simulink model "ME655_project"  (R2023b)
settings: Solver=FixedStepAuto  StartTime=0.0  StopTime=60.0  FixedStep=.003  RelTol=1e-3
values from neighbouring files (symbols this model uses):
  A = [1 T; 0 1]    [ME655_project_Matlab_code.m]
  dt_active_control = 10    [ME655_project_Matlab_code.m]
  H = eye(2)    [ME655_project_Matlab_code.m]
  h = 2.5*N    (= 200)    [ME655_project_Matlab_code.m]
  K = Sp * C * inv(Sh)    [ME655_project_Matlab_code.m]
  k = -K * RhipAvg' + LhipAvg'    [ME655_project_Matlab_code.m]
  lambda = .95    (= 0.95)    [ME655_project_Matlab_code.m]
  Lhip_pos0 = Lhip_pos(1)    [ME655_project_Matlab_code.m]
  Lhip_vel0 = Lhip_vel(1)    [ME655_project_Matlab_code.m]
  M = 6    [ME655_project_Matlab_code.m]
  N = 80    [ME655_project_Matlab_code.m]
  nu = .5    (= 0.5)    [ME655_project_Matlab_code.m]
  Q = G * G' * var(Lhip_acc(train_indices))    [ME655_project_Matlab_code.m]
  R = diag([var(Lhip_pred(:, 1) - Lhip_pos_train), var(Lhip_pred(:, 2) - Lhip_vel_train)])    [ME655_project_Matlab_code.m]
  t_start = 5.0    (= 5)    [ME655_project_Matlab_code.m]
  Tau_h_max = 30    [ME655_project_Matlab_code.m]
undefined symbols (not defined in the file or in its folder): Bh, g, IHC, IRC, Kh, LH, LR, mH, mR, theta_0, theta_d0
settings Model: Creator=Damiano  LastModifiedBy=Mihir
settings SolverCC: AlgebraicLoopSolver=TrustRegion
settings DataIOCC: ReturnWorkspaceOutputs=off
settings DebuggingCC: UnconnectedInputMsg=warning  UnconnectedOutputMsg=warning  UnconnectedLineMsg=warning  ArithmeticOperatorsInVariantConditions=warning
settings ModelReferenceCC: EnableRefExpFcnMdlSchedulingChecks=on
settings SFSimCC: SimUseLocalCustomCode=off  CustomCodeUndefinedFunction=UseInterfaceOnly
settings RTWCC: RTWUseLocalCustomCode=off  DLArmComputeVersion=19.05
settings CodeAppCC: StateflowObjectComments=on

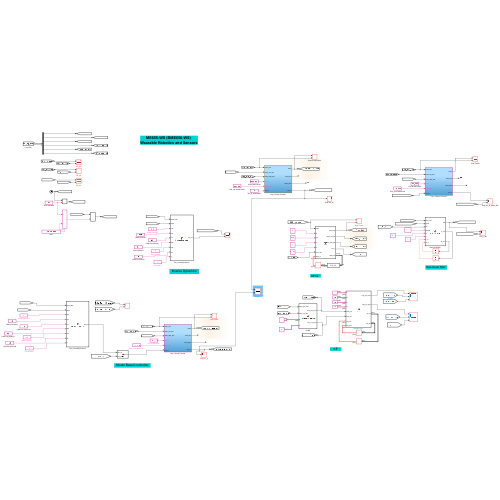
[thumbnail: Simulink's stored preview of the top-level diagram]
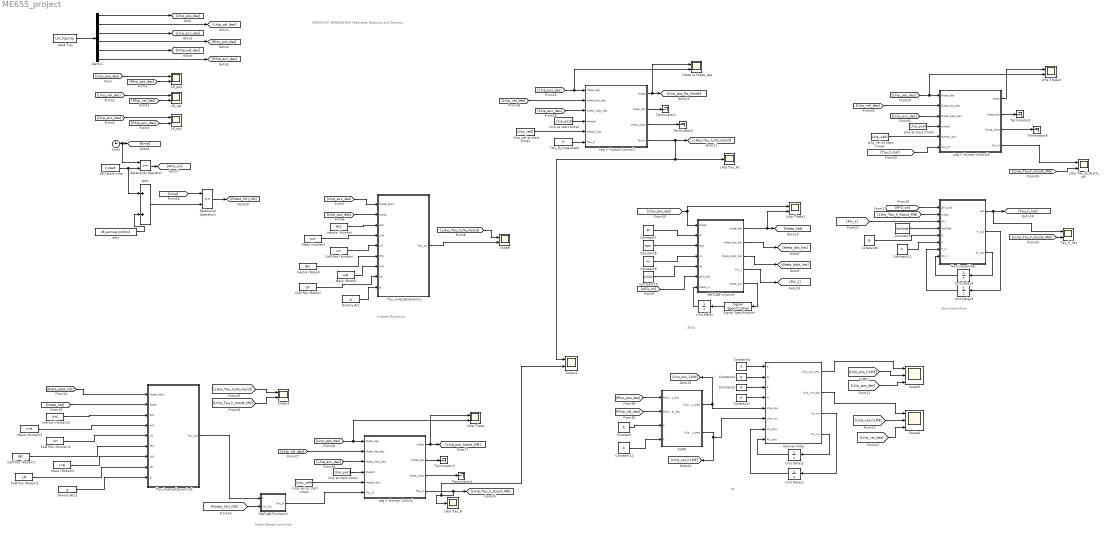
== system ME655_project ==
  note: ME655-WS (BME656-WS)
      | Wearable Robotics and Sensors
  note: AFOs
  note: Inverse Dynamics
  note: Model Based controller
  note: KF
  note: Non-linear filter
  AFO start time : Constant  Value=t_start
  Add : Sum
  CLME : MATLAB Function  TreatAsAtomicUnit=on
  Clock : Clock
  CoM Pos (Human) : Constant  Value=LH
  CoM Pos (Human)2 : Constant  Value=LH
  CoM Pos (Robot) : Constant  Value=LR
  CoM Pos (Robot)1 : Constant  Value=IRC
  CoM Pos (Robot)2 : Constant  Value=LR
  Constant : Constant  Value=K
  Constant1 : Constant  Value=H
  Constant10 : Constant  Value=0.003
  Constant11 : Constant  Value=h
  Constant12 : Constant  Value=k
  Constant2 : Constant  Value=R
  Constant3 : Constant  Value=Q
  Constant4 : Constant  Value=A
  Constant5 : Constant  Value=lambda
  Constant6 : Constant  Value=N
  Constant7 : Constant  Value=M
  Constant8 : Constant  Value=eps
  Constant9 : Constant  Value=nu
  Demux : Demux  Outputs=6
  Gravity Acc : Constant  Value=g
  Gravity Acc2 : Constant  Value=g
  Inertia (Human) : Constant  Value=IHC
  Inertia (Human)2 : Constant  Value=IHC
  Inertia (Robot) : Constant  Value=IRC
  Kalman Filter : MATLAB Function  TreatAsAtomicUnit=on
  LHip Tau_H : Scope
  LHip Tau_H1 : Scope
  LHip Tau_H_Assist_MF : Scope  NumInputPorts=2
  LHip Theta : Scope  NumInputPorts=2
  LHip Theta1 : Scope  NumInputPorts=2
  LHip Theta3 : Scope  NumInputPorts=2
  "LR_acc " : Scope  NumInputPorts=2
  LR_pos : Scope  NumInputPorts=2
  LR_vel : Scope  NumInputPorts=2
  Leg + Human Control : Subsystem
  Leg + Human Control1 : Subsystem
  Leg + Human Control2 : Subsystem
  Lhip at start time1 : Constant  Value=Lhip_pos0
  Lhip at start time2 : Constant  Value=Lhip_pos0
  Lhip at start time3 : Constant  Value=Lhip_pos0
  Lhip_vel at start time1 : Constant  Value=Lhip_vel0
  Lhip_vel at start time2 : Constant  Value=Lhip_vel0
  Lhip_vel at start time3 : Constant  Value=Lhip_vel0
  Load Traj : FromWorkspace  VariableName=LH_hip_traj
  MATLAB Function : MATLAB Function  TreatAsAtomicUnit=on
  MATLAB Function1 : MATLAB Function  TreatAsAtomicUnit=on
  Mass (Human) : Constant  Value=mH
  Mass (Human)2 : Constant  Value=mH
  Mass (Robot) : Constant  Value=mR
  Mass (Robot)2 : Constant  Value=mR
  NonLinearFilter : MATLAB Function  TreatAsAtomicUnit=on
  Relational Operator : RelationalOperator  OutDataTypeStr=boolean  RndMeth=Simplest  InputSameDT=off
  Relational Operator1 : RelationalOperator  OutDataTypeStr=boolean  RndMeth=Simplest  InputSameDT=off
  Scope : Scope  NumInputPorts=2
  Scope1 : Scope  NumInputPorts=2
  Scope3 : Scope  NumInputPorts=2
  Scope5 : Scope  NumInputPorts=3
  Scope6 : Scope  NumInputPorts=3
  Signal Specification : SignalSpecification  Dimensions=[1,14]
  Tau_InverseDynamics : MATLAB Function  TreatAsAtomicUnit=on
  Tau_InverseDynamics2 : MATLAB Function  TreatAsAtomicUnit=on
  Tau_R_Unassisted : Constant  Value=0
  Tau_h_hat : Scope  NumInputPorts=2
  Terminator{1..6} (6 alike) : Terminator
  Unit Delay : UnitDelay  InitialCondition=[[pi/2,pi/2,pi/2,pi/2,pi/2,pi/2],[0,0,0,0,0,0], 3*pi/2, 0]  SampleTime=-1  HasFrameUpgradeWarning=on
  Unit Delay1 : UnitDelay  InitialCondition=eye(2)  SampleTime=-1  HasFrameUpgradeWarning=on
  Unit Delay2 : UnitDelay  InitialCondition=[0;0]  SampleTime=-1  HasFrameUpgradeWarning=on
  Unit Delay3 : UnitDelay  InitialCondition=1  SampleTime=-1  HasFrameUpgradeWarning=on
  Unit Delay4 : UnitDelay  SampleTime=-1  HasFrameUpgradeWarning=on
  theta vs theta_des : Scope  NumInputPorts=2
  zero : Constant  Value=dt_active_control
  wires:
  Load Traj/1 -> Demux/1
  Demux/6 -> [Rhip_acc_des]
  Demux/4 -> [Rhip_pos_des]
  Demux/5 -> [Rhip_vel_des]
  [Lhip_pos_des] -> LR_pos/1
  [Rhip_pos_des] -> LR_pos/2
  [Lhip_vel_des] -> LR_vel/1
  [Rhip_vel_des] -> LR_vel/2
  [Lhip_acc_des] -> "LR_acc "/1
  [Rhip_acc_des] -> "LR_acc "/2
  Clock/1 -> Relational Operator/1, [time]
  Relational Operator/1 -> [AFO_on]
  [time] -> Relational Operator1/1
  AFO start time/1 -> Add/1, Relational Operator/2
  Add/1 -> Relational Operator1/2
  zero/1 -> Add/2
  [Lhip_acc_des] -> Leg + Human Control/3(theta_ddot_des)
  Leg + Human Control/3(theta_ddot) -> Terminator4/1
  Lhip_vel at start time1/1 -> Leg + Human Control/5(theta0_dot)
  Leg + Human Control/2(theta_dot) -> Terminator3/1
  [Lhip_vel_des] -> Leg + Human Control/2(theta_dot_des)
  Lhip at start time1/1 -> Leg + Human Control/4(theta0)
  Leg + Human Control/1(theta) -> LHip Theta/1, [Lhip_pos_Assist_MB]
  Leg + Human Control/4(Tau_h) -> Scope1/2, LHip Tau_H/1, [LHip_Tau_h_Assist_MB]
  [Lhip_pos_des] -> Leg + Human Control/1(theta_des), LHip Theta/2
  Relational Operator1/1 -> [Robot_Ctrl_ON]
  Demux/1 -> [Lhip_pos_des]
  Demux/2 -> [Lhip_vel_des]
  Demux/3 -> [Lhip_acc_des]
  Inertia (Robot)/1 -> Tau_InverseDynamics/6(IRC)
  Gravity Acc/1 -> Tau_InverseDynamics/9(g)
  Mass (Robot)/1 -> Tau_InverseDynamics/7(mR)
  Inertia (Human)/1 -> Tau_InverseDynamics/3(IHC)
  Mass (Human)/1 -> Tau_InverseDynamics/4(mH)
  CoM Pos (Robot)/1 -> Tau_InverseDynamics/8(LR)
  CoM Pos (Human)/1 -> Tau_InverseDynamics/5(LH)
  [Lhip_pos_des] -> Tau_InverseDynamics/2(theta)
  [Lhip_acc_des] -> Tau_InverseDynamics/1(theta_ddot)
  [LHip_Tau_h_No_Assist] -> Scope/1
  MATLAB Function/2(theta_dot_hat) -> [theta_dot_hat]
  MATLAB Function/1(theta_hat) -> [theta_hat], LHip Theta1/2
  MATLAB Function/3(theta_ddot_hat) -> [theta_ddot_hat]
  [AFO_on] -> MATLAB Function/6(AFO_ON)
  Signal Specification/1 -> Unit Delay/1
  [Lhip_pos_des] -> LHip Theta1/1, MATLAB Function/1(theta)
  Constant7/1 -> MATLAB Function/2(M)
  Constant8/1 -> MATLAB Function/3(eps)
  Constant10/1 -> MATLAB Function/5(dt)
  Constant9/1 -> MATLAB Function/4(nu)
  Tau_InverseDynamics/1(Tau_tot) -> Scope/2
  MATLAB Function/5(state_out) -> Signal Specification/1
  Unit Delay/1 -> MATLAB Function/7(state_in)
  [LHip_Tau_h_Assist_MB] -> Scope3/2
  Mass (Robot)2/1 -> Tau_InverseDynamics2/7(mR)
  Tau_InverseDynamics2/1(Tau_tot) -> MATLAB Function1/1(Tau_tot)
  Mass (Human)2/1 -> Tau_InverseDynamics2/4(mH)
  Gravity Acc2/1 -> Tau_InverseDynamics2/9(g)
  Inertia (Human)2/1 -> Tau_InverseDynamics2/3(IHC)
  [theta_hat] -> Tau_InverseDynamics2/2(theta)
  CoM Pos (Human)2/1 -> Tau_InverseDynamics2/5(LH)
  [theta_ddot_hat] -> Tau_InverseDynamics2/1(theta_ddot)
  CoM Pos (Robot)2/1 -> Tau_InverseDynamics2/8(LR)
  CoM Pos (Robot)1/1 -> Tau_InverseDynamics2/6(IRC)
  [LHip_Tau_h_No_Assist] -> Scope3/1
  Constant2/1 -> Kalman Filter/3(R)
  Constant3/1 -> Kalman Filter/2(Q)
  Constant4/1 -> Kalman Filter/1(A)
  Kalman Filter/2(Lhip_vel_des) -> Scope6/1
  Kalman Filter/4(Pk_nxt) -> Unit Delay1/1
  Kalman Filter/1(Lhip_pos_des) -> Scope5/1
  Unit Delay2/1 -> Kalman Filter/7(xk_prev)
  [Lhip_vel_des] -> Scope6/3
  [Lhip_pos_CLME] -> Scope5/2
  [Lhip_vel_CLME] -> Scope6/2
  [Lhip_pos_des] -> Scope5/3
  Constant1/1 -> Kalman Filter/4(H)
  Kalman Filter/3(xk_nxt) -> Unit Delay2/1
  Unit Delay1/1 -> Kalman Filter/8(Pk_prev)
  MATLAB Function1/1(Tau_R) -> Leg + Human Control/6(Tau_R)
  Leg + Human Control1/3(theta_ddot) -> Terminator2/1
  Leg + Human Control1/2(theta_dot) -> Terminator1/1
  [Lhip_pos_des] -> Leg + Human Control1/1(theta_des), theta vs theta_des/2
  [Lhip_vel_des] -> Leg + Human Control1/2(theta_dot_des)
  Lhip_vel at start time2/1 -> Leg + Human Control1/5(theta0_dot)
  Leg + Human Control1/4(Tau_h) -> LHip Tau_H1/1, Scope1/1, [LHip_Tau_h_No_Assist]
  Lhip at start time2/1 -> Leg + Human Control1/4(theta0)
  Tau_R_Unassisted/1 -> Leg + Human Control1/6(Tau_R)
  [Lhip_acc_des] -> Leg + Human Control1/3(theta_ddot_des)
  Leg + Human Control1/1(theta) -> theta vs theta_des/1, [Lhip_pos_No_Assist]
  [Robot_Ctrl_ON] -> MATLAB Function1/2(Ctrl_On)
  MATLAB Function/4(Phi_1) -> [Phi_1]
  NonLinearFilter/1(est) -> Tau_h_hat/1, [Tau_h_hat]
  NonLinearFilter/3(W_out) -> Unit Delay4/1
  [AFO_on] -> NonLinearFilter/1(AFO_ON)
  Unit Delay4/1 -> NonLinearFilter/8(W_in)
  Constant11/1 -> NonLinearFilter/6(h)
  NonLinearFilter/2(P_out) -> Unit Delay3/1
  Constant6/1 -> NonLinearFilter/5(N)
  Unit Delay3/1 -> NonLinearFilter/7(P_in)
  Constant5/1 -> NonLinearFilter/4(lambda)
  [LHip_Tau_h_Assist_MB] -> NonLinearFilter/2(meas)
  [Phi_1] -> NonLinearFilter/3(phi)
  [Lhip_vel_des] -> Leg + Human Control2/2(theta_dot_des)
  Leg + Human Control2/2(theta_dot) -> Terminator5/1
  [Lhip_acc_des] -> Leg + Human Control2/3(theta_ddot_des)
  Leg + Human Control2/1(theta) -> LHip Theta3/1
  Lhip_vel at start time3/1 -> Leg + Human Control2/5(theta0_dot)
  Lhip at start time3/1 -> Leg + Human Control2/4(theta0)
  Leg + Human Control2/4(Tau_h) -> LHip Tau_H_Assist_MF/1
  [Tau_h_hat] -> Leg + Human Control2/6(Tau_R)
  Leg + Human Control2/3(theta_ddot) -> Terminator6/1
  [Lhip_pos_des] -> Leg + Human Control2/1(theta_des), LHip Theta3/2
  [LHip_Tau_h_Assist_MB] -> LHip Tau_H_Assist_MF/2
  [Rhip_vel_des] -> CLME/2(Rhip_vel_des)
  [Rhip_pos_des] -> CLME/1(Rhip_pos_des)
  Constant/1 -> CLME/3(K)
  Constant12/1 -> CLME/4(k)
  CLME/1(Lhip_pos_pred) -> [Lhip_pos_CLME], Kalman Filter/5(Lhip_pos)
  CLME/2(Lhip_vel_pred) -> [Lhip_vel_CLME], Kalman Filter/6(Lhip_vel)
  [LHip_Tau_h_Assist_MB] -> Tau_h_hat/2

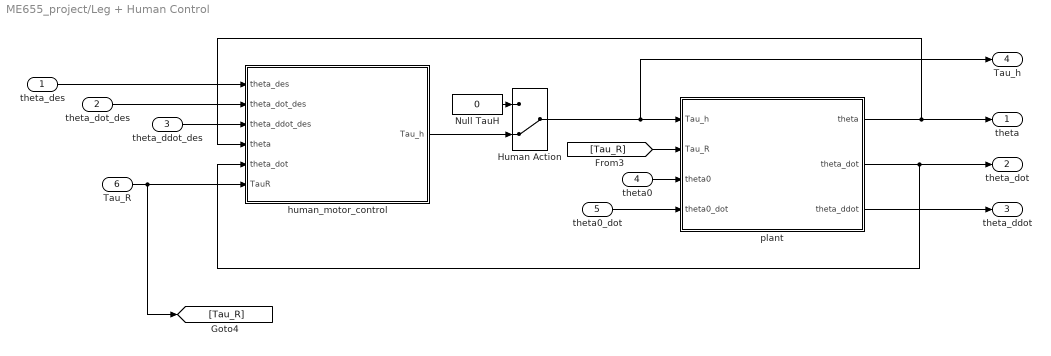
== system ME655_project/Leg + Human Control ==
  theta_des : Inport
  theta_dot_des : Inport  Port=2
  theta_ddot_des : Inport  Port=3
  theta0 : Inport  Port=4
  theta0_dot : Inport  Port=5
  Tau_R : Inport  Port=6
  Human Action : ManualSwitch  CurrentSetting=0
  Null TauH : Constant  Value=0
  human_motor_control : Subsystem
  plant : Subsystem
  theta : Outport  PortDimensions=[1,1]  VectorParamsAs1DForOutWhenUnconnected=off
  theta_dot : Outport  Port=2  PortDimensions=[1,1]  VectorParamsAs1DForOutWhenUnconnected=off
  theta_ddot : Outport  Port=3  PortDimensions=[1,1]  VectorParamsAs1DForOutWhenUnconnected=off
  Tau_h : Outport  Port=4  PortDimensions=[1,1]  VectorParamsAs1DForOutWhenUnconnected=off
  wires:
  theta_des/1 -> human_motor_control/1(theta_des)
  theta_dot_des/1 -> human_motor_control/2(theta_dot_des)
  theta0/1 -> plant/3(theta0)
  theta0_dot/1 -> plant/4(theta0_dot)
  [Tau_R] -> plant/2(Tau_R)
  plant/1(theta) -> theta/1, human_motor_control/4(theta)
  plant/2(theta_dot) -> human_motor_control/5(theta_dot), theta_dot/1
  plant/3(theta_ddot) -> theta_ddot/1
  theta_ddot_des/1 -> human_motor_control/3(theta_ddot_des)
  human_motor_control/1(Tau_h) -> Human Action/2
  Human Action/1 -> Tau_h/1, plant/1(Tau_h)
  Null TauH/1 -> Human Action/1
  Tau_R/1 -> [Tau_R], human_motor_control/6(TauR)

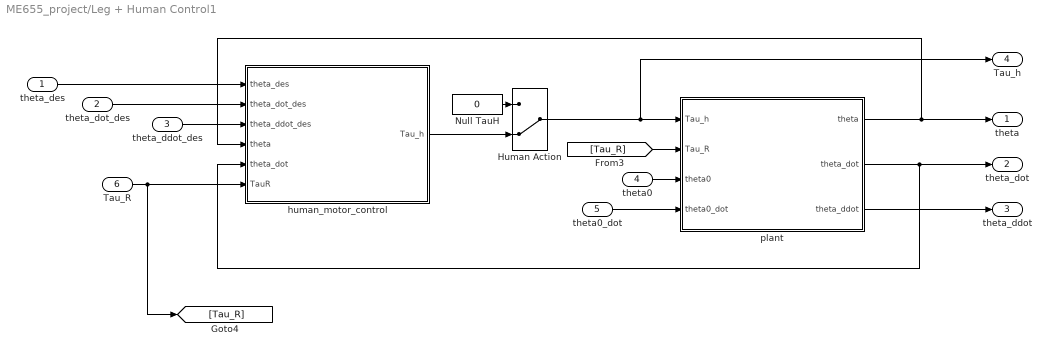
== system ME655_project/Leg + Human Control1 ==
  theta_des : Inport
  theta_dot_des : Inport  Port=2
  theta_ddot_des : Inport  Port=3
  theta0 : Inport  Port=4
  theta0_dot : Inport  Port=5
  Tau_R : Inport  Port=6
  Human Action : ManualSwitch  CurrentSetting=0
  Null TauH : Constant  Value=0
  human_motor_control : Subsystem
  plant : Subsystem
  theta : Outport  PortDimensions=[1,1]  VectorParamsAs1DForOutWhenUnconnected=off
  theta_dot : Outport  Port=2  PortDimensions=[1,1]  VectorParamsAs1DForOutWhenUnconnected=off
  theta_ddot : Outport  Port=3  PortDimensions=[1,1]  VectorParamsAs1DForOutWhenUnconnected=off
  Tau_h : Outport  Port=4  PortDimensions=[1,1]  VectorParamsAs1DForOutWhenUnconnected=off
  wires:
  theta_des/1 -> human_motor_control/1(theta_des)
  theta_dot_des/1 -> human_motor_control/2(theta_dot_des)
  theta0/1 -> plant/3(theta0)
  theta0_dot/1 -> plant/4(theta0_dot)
  [Tau_R] -> plant/2(Tau_R)
  plant/1(theta) -> theta/1, human_motor_control/4(theta)
  plant/2(theta_dot) -> human_motor_control/5(theta_dot), theta_dot/1
  plant/3(theta_ddot) -> theta_ddot/1
  theta_ddot_des/1 -> human_motor_control/3(theta_ddot_des)
  human_motor_control/1(Tau_h) -> Human Action/2
  Human Action/1 -> Tau_h/1, plant/1(Tau_h)
  Null TauH/1 -> Human Action/1
  Tau_R/1 -> [Tau_R], human_motor_control/6(TauR)

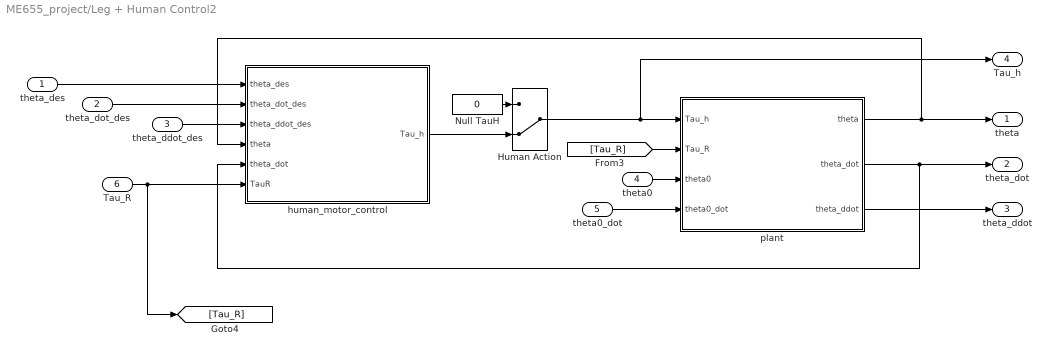
== system ME655_project/Leg + Human Control2 ==
  theta_des : Inport
  theta_dot_des : Inport  Port=2
  theta_ddot_des : Inport  Port=3
  theta0 : Inport  Port=4
  theta0_dot : Inport  Port=5
  Tau_R : Inport  Port=6
  Human Action : ManualSwitch  CurrentSetting=0
  Null TauH : Constant  Value=0
  human_motor_control : Subsystem
  plant : Subsystem
  theta : Outport  PortDimensions=[1,1]  VectorParamsAs1DForOutWhenUnconnected=off
  theta_dot : Outport  Port=2  PortDimensions=[1,1]  VectorParamsAs1DForOutWhenUnconnected=off
  theta_ddot : Outport  Port=3  PortDimensions=[1,1]  VectorParamsAs1DForOutWhenUnconnected=off
  Tau_h : Outport  Port=4  PortDimensions=[1,1]  VectorParamsAs1DForOutWhenUnconnected=off
  wires:
  theta_des/1 -> human_motor_control/1(theta_des)
  theta_dot_des/1 -> human_motor_control/2(theta_dot_des)
  theta0/1 -> plant/3(theta0)
  theta0_dot/1 -> plant/4(theta0_dot)
  [Tau_R] -> plant/2(Tau_R)
  plant/1(theta) -> theta/1, human_motor_control/4(theta)
  plant/2(theta_dot) -> human_motor_control/5(theta_dot), theta_dot/1
  plant/3(theta_ddot) -> theta_ddot/1
  theta_ddot_des/1 -> human_motor_control/3(theta_ddot_des)
  human_motor_control/1(Tau_h) -> Human Action/2
  Human Action/1 -> Tau_h/1, plant/1(Tau_h)
  Null TauH/1 -> Human Action/1
  Tau_R/1 -> [Tau_R], human_motor_control/6(TauR)

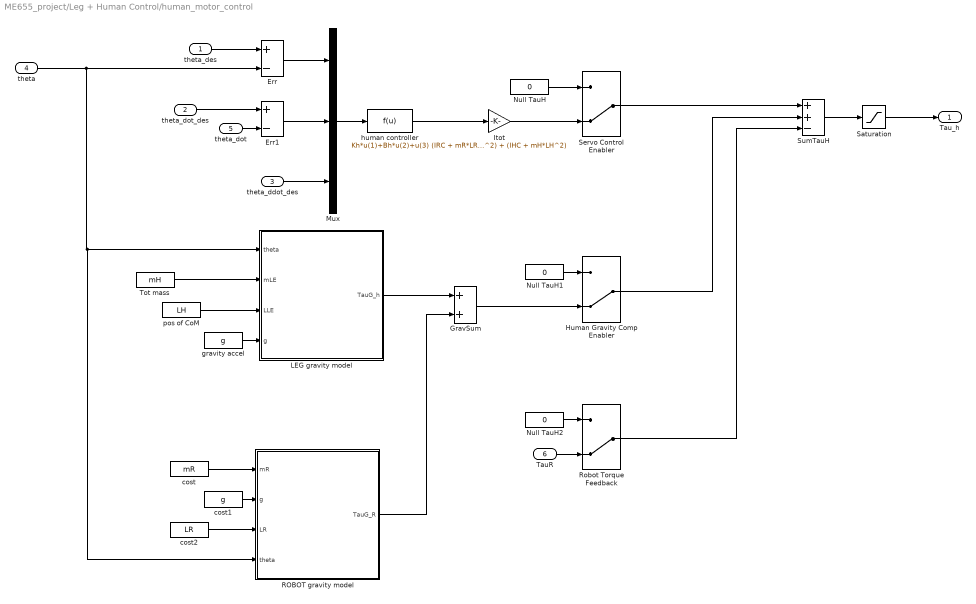
== system ME655_project/Leg + Human Control/human_motor_control ==
  theta_des : Inport
  theta_dot_des : Inport  Port=2
  theta_ddot_des : Inport  Port=3
  theta : Inport  Port=4
  theta_dot : Inport  Port=5
  TauR : Inport  Port=6
  Err : Sum  Inputs=+-
  Err1 : Sum  Inputs=+-
  GravSum : Sum
  Human Gravity Comp Enabler : ManualSwitch  CurrentSetting=0
  Itot : Gain  Gain=(IRC + mR*LR^2) + (IHC + mH*LH^2)
  LEG gravity model : MATLAB Function  TreatAsAtomicUnit=on
  Mux : Mux  Inputs=3
  Null TauH : Constant  Value=0
  Null TauH1 : Constant  Value=0
  Null TauH2 : Constant  Value=0
  ROBOT gravity model : MATLAB Function  TreatAsAtomicUnit=on
  Robot Torque Feedback : ManualSwitch  CurrentSetting=0
  Saturation : Saturate  UpperLimit=Tau_h_max  LowerLimit=-Tau_h_max
  Servo Control Enabler : ManualSwitch  CurrentSetting=0
  SumTauH : Sum  Inputs=++-
  Tot mass : Constant  Value=mH
  cost : Constant  Value=mR
  cost1 : Constant  Value=g
  cost2 : Constant  Value=LR
  gravity accel : Constant  Value=g
  human controller : Fcn  Expr=Kh*u(1)+Bh*u(2)+u(3)
  pos of CoM : Constant  Value=LH
  Tau_h : Outport  PortDimensions=[1,1]  VectorParamsAs1DForOutWhenUnconnected=off
  wires:
  theta_des/1 -> Err/1
  theta_dot_des/1 -> Err1/1
  theta_dot/1 -> Err1/2
  Err/1 -> Mux/1
  Err1/1 -> Mux/2
  Mux/1 -> human controller/1
  theta_ddot_des/1 -> Mux/3
  gravity accel/1 -> LEG gravity model/4(g)
  Tot mass/1 -> LEG gravity model/2(mLE)
  pos of CoM/1 -> LEG gravity model/3(LLE)
  Null TauH/1 -> Servo Control Enabler/1
  Null TauH1/1 -> Human Gravity Comp Enabler/1
  Human Gravity Comp Enabler/1 -> SumTauH/2
  SumTauH/1 -> Saturation/1
  human controller/1 -> Itot/1
  Servo Control Enabler/1 -> SumTauH/1
  Saturation/1 -> Tau_h/1
  Itot/1 -> Servo Control Enabler/2
  Null TauH2/1 -> Robot Torque Feedback/1
  TauR/1 -> Robot Torque Feedback/2
  Robot Torque Feedback/1 -> SumTauH/3
  theta/1 -> ROBOT gravity model/4(theta), LEG gravity model/1(theta), Err/2
  ROBOT gravity model/1(TauG_R) -> GravSum/2
  cost2/1 -> ROBOT gravity model/3(LR)
  cost/1 -> ROBOT gravity model/1(mR)
  cost1/1 -> ROBOT gravity model/2(g)
  LEG gravity model/1(TauG_h) -> GravSum/1
  GravSum/1 -> Human Gravity Comp Enabler/2

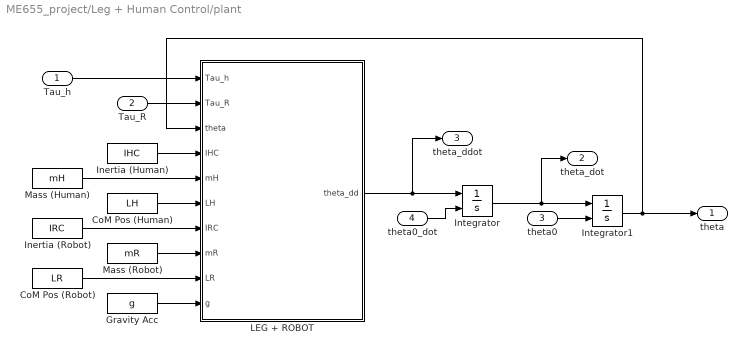
== system ME655_project/Leg + Human Control/plant ==
  Tau_h : Inport
  Tau_R : Inport  Port=2
  theta0 : Inport  Port=3
  theta0_dot : Inport  Port=4
  CoM Pos (Human) : Constant  Value=LH
  CoM Pos (Robot) : Constant  Value=LR
  Gravity Acc : Constant  Value=g
  Inertia (Human) : Constant  Value=IHC
  Inertia (Robot) : Constant  Value=IRC
  Integrator : Integrator  InitialConditionSource=external  InitialCondition=theta_d0
  Integrator1 : Integrator  InitialConditionSource=external  InitialCondition=theta_0
  LEG + ROBOT : MATLAB Function  TreatAsAtomicUnit=on
  Mass (Human) : Constant  Value=mH
  Mass (Robot) : Constant  Value=mR
  theta : Outport  PortDimensions=[1,1]  VectorParamsAs1DForOutWhenUnconnected=off
  theta_dot : Outport  Port=2  PortDimensions=[1,1]  VectorParamsAs1DForOutWhenUnconnected=off
  theta_ddot : Outport  Port=3  PortDimensions=[1,1]  VectorParamsAs1DForOutWhenUnconnected=off
  wires:
  Tau_h/1 -> LEG + ROBOT/1(Tau_h)
  Tau_R/1 -> LEG + ROBOT/2(Tau_R)
  LEG + ROBOT/1(theta_dd) -> theta_ddot/1, Integrator/1
  Integrator/1 -> theta_dot/1, Integrator1/1
  theta0_dot/1 -> Integrator/2
  theta0/1 -> Integrator1/2
  Integrator1/1 -> LEG + ROBOT/3(theta), theta/1
  Inertia (Human)/1 -> LEG + ROBOT/4(IHC)
  Mass (Human)/1 -> LEG + ROBOT/5(mH)
  CoM Pos (Human)/1 -> LEG + ROBOT/6(LH)
  Gravity Acc/1 -> LEG + ROBOT/10(g)
  Mass (Robot)/1 -> LEG + ROBOT/8(mR)
  CoM Pos (Robot)/1 -> LEG + ROBOT/9(LR)
  Inertia (Robot)/1 -> LEG + ROBOT/7(IRC)

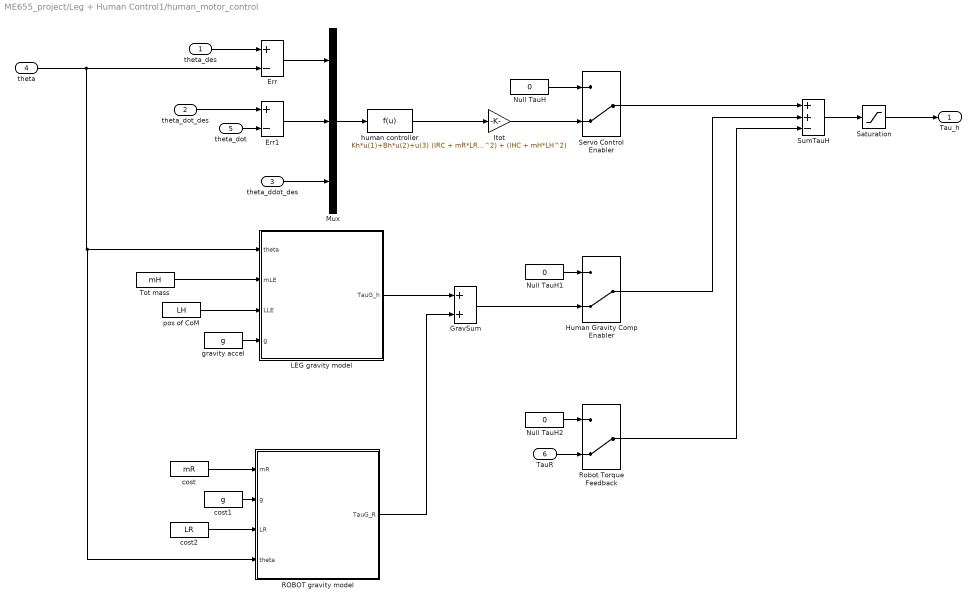
== system ME655_project/Leg + Human Control1/human_motor_control ==
  theta_des : Inport
  theta_dot_des : Inport  Port=2
  theta_ddot_des : Inport  Port=3
  theta : Inport  Port=4
  theta_dot : Inport  Port=5
  TauR : Inport  Port=6
  Err : Sum  Inputs=+-
  Err1 : Sum  Inputs=+-
  GravSum : Sum
  Human Gravity Comp Enabler : ManualSwitch  CurrentSetting=0
  Itot : Gain  Gain=(IRC + mR*LR^2) + (IHC + mH*LH^2)
  LEG gravity model : MATLAB Function  TreatAsAtomicUnit=on
  Mux : Mux  Inputs=3
  Null TauH : Constant  Value=0
  Null TauH1 : Constant  Value=0
  Null TauH2 : Constant  Value=0
  ROBOT gravity model : MATLAB Function  TreatAsAtomicUnit=on
  Robot Torque Feedback : ManualSwitch  CurrentSetting=0
  Saturation : Saturate  UpperLimit=Tau_h_max  LowerLimit=-Tau_h_max
  Servo Control Enabler : ManualSwitch  CurrentSetting=0
  SumTauH : Sum  Inputs=++-
  Tot mass : Constant  Value=mH
  cost : Constant  Value=mR
  cost1 : Constant  Value=g
  cost2 : Constant  Value=LR
  gravity accel : Constant  Value=g
  human controller : Fcn  Expr=Kh*u(1)+Bh*u(2)+u(3)
  pos of CoM : Constant  Value=LH
  Tau_h : Outport  PortDimensions=[1,1]  VectorParamsAs1DForOutWhenUnconnected=off
  wires:
  theta_des/1 -> Err/1
  theta_dot_des/1 -> Err1/1
  theta_dot/1 -> Err1/2
  Err/1 -> Mux/1
  Err1/1 -> Mux/2
  Mux/1 -> human controller/1
  theta_ddot_des/1 -> Mux/3
  gravity accel/1 -> LEG gravity model/4(g)
  Tot mass/1 -> LEG gravity model/2(mLE)
  pos of CoM/1 -> LEG gravity model/3(LLE)
  Null TauH/1 -> Servo Control Enabler/1
  Null TauH1/1 -> Human Gravity Comp Enabler/1
  Human Gravity Comp Enabler/1 -> SumTauH/2
  SumTauH/1 -> Saturation/1
  human controller/1 -> Itot/1
  Servo Control Enabler/1 -> SumTauH/1
  Saturation/1 -> Tau_h/1
  Itot/1 -> Servo Control Enabler/2
  Null TauH2/1 -> Robot Torque Feedback/1
  TauR/1 -> Robot Torque Feedback/2
  Robot Torque Feedback/1 -> SumTauH/3
  theta/1 -> ROBOT gravity model/4(theta), LEG gravity model/1(theta), Err/2
  ROBOT gravity model/1(TauG_R) -> GravSum/2
  cost2/1 -> ROBOT gravity model/3(LR)
  cost/1 -> ROBOT gravity model/1(mR)
  cost1/1 -> ROBOT gravity model/2(g)
  LEG gravity model/1(TauG_h) -> GravSum/1
  GravSum/1 -> Human Gravity Comp Enabler/2

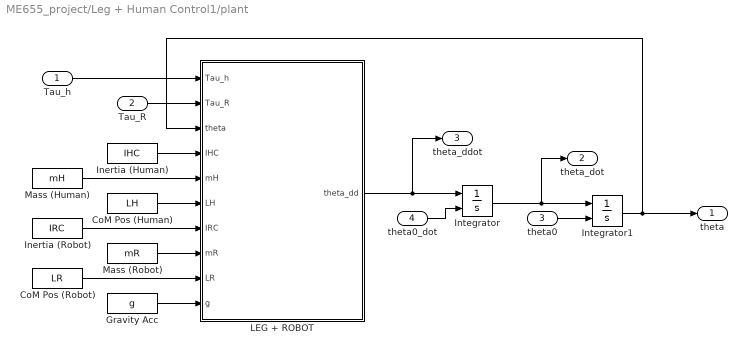
== system ME655_project/Leg + Human Control1/plant ==
  Tau_h : Inport
  Tau_R : Inport  Port=2
  theta0 : Inport  Port=3
  theta0_dot : Inport  Port=4
  CoM Pos (Human) : Constant  Value=LH
  CoM Pos (Robot) : Constant  Value=LR
  Gravity Acc : Constant  Value=g
  Inertia (Human) : Constant  Value=IHC
  Inertia (Robot) : Constant  Value=IRC
  Integrator : Integrator  InitialConditionSource=external  InitialCondition=theta_d0
  Integrator1 : Integrator  InitialConditionSource=external  InitialCondition=theta_0
  LEG + ROBOT : MATLAB Function  TreatAsAtomicUnit=on
  Mass (Human) : Constant  Value=mH
  Mass (Robot) : Constant  Value=mR
  theta : Outport  PortDimensions=[1,1]  VectorParamsAs1DForOutWhenUnconnected=off
  theta_dot : Outport  Port=2  PortDimensions=[1,1]  VectorParamsAs1DForOutWhenUnconnected=off
  theta_ddot : Outport  Port=3  PortDimensions=[1,1]  VectorParamsAs1DForOutWhenUnconnected=off
  wires:
  Tau_h/1 -> LEG + ROBOT/1(Tau_h)
  Tau_R/1 -> LEG + ROBOT/2(Tau_R)
  LEG + ROBOT/1(theta_dd) -> theta_ddot/1, Integrator/1
  Integrator/1 -> theta_dot/1, Integrator1/1
  theta0_dot/1 -> Integrator/2
  theta0/1 -> Integrator1/2
  Integrator1/1 -> LEG + ROBOT/3(theta), theta/1
  Inertia (Human)/1 -> LEG + ROBOT/4(IHC)
  Mass (Human)/1 -> LEG + ROBOT/5(mH)
  CoM Pos (Human)/1 -> LEG + ROBOT/6(LH)
  Gravity Acc/1 -> LEG + ROBOT/10(g)
  Mass (Robot)/1 -> LEG + ROBOT/8(mR)
  CoM Pos (Robot)/1 -> LEG + ROBOT/9(LR)
  Inertia (Robot)/1 -> LEG + ROBOT/7(IRC)

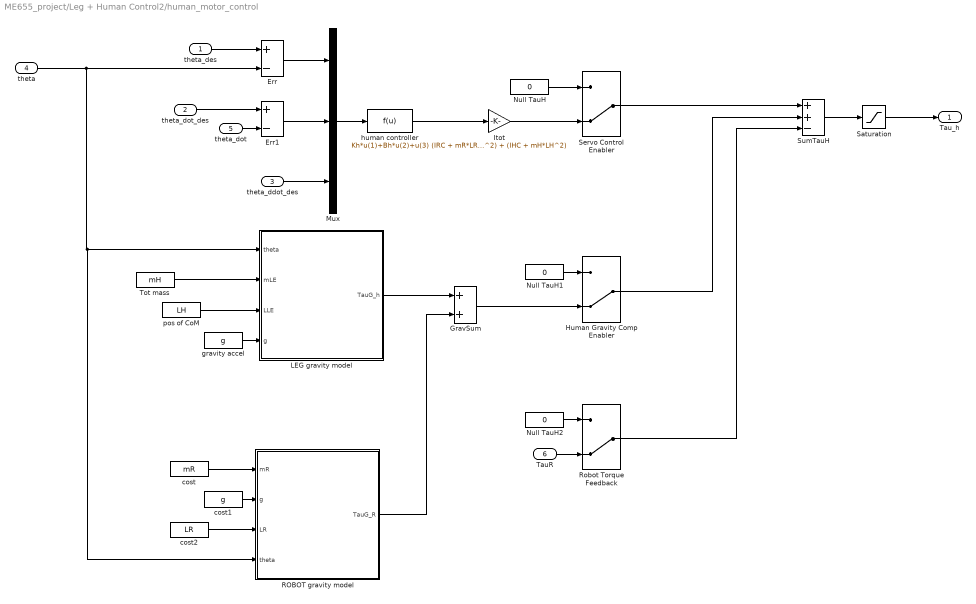
== system ME655_project/Leg + Human Control2/human_motor_control ==
  theta_des : Inport
  theta_dot_des : Inport  Port=2
  theta_ddot_des : Inport  Port=3
  theta : Inport  Port=4
  theta_dot : Inport  Port=5
  TauR : Inport  Port=6
  Err : Sum  Inputs=+-
  Err1 : Sum  Inputs=+-
  GravSum : Sum
  Human Gravity Comp Enabler : ManualSwitch  CurrentSetting=0
  Itot : Gain  Gain=(IRC + mR*LR^2) + (IHC + mH*LH^2)
  LEG gravity model : MATLAB Function  TreatAsAtomicUnit=on
  Mux : Mux  Inputs=3
  Null TauH : Constant  Value=0
  Null TauH1 : Constant  Value=0
  Null TauH2 : Constant  Value=0
  ROBOT gravity model : MATLAB Function  TreatAsAtomicUnit=on
  Robot Torque Feedback : ManualSwitch  CurrentSetting=0
  Saturation : Saturate  UpperLimit=Tau_h_max  LowerLimit=-Tau_h_max
  Servo Control Enabler : ManualSwitch  CurrentSetting=0
  SumTauH : Sum  Inputs=++-
  Tot mass : Constant  Value=mH
  cost : Constant  Value=mR
  cost1 : Constant  Value=g
  cost2 : Constant  Value=LR
  gravity accel : Constant  Value=g
  human controller : Fcn  Expr=Kh*u(1)+Bh*u(2)+u(3)
  pos of CoM : Constant  Value=LH
  Tau_h : Outport  PortDimensions=[1,1]  VectorParamsAs1DForOutWhenUnconnected=off
  wires:
  theta_des/1 -> Err/1
  theta_dot_des/1 -> Err1/1
  theta_dot/1 -> Err1/2
  Err/1 -> Mux/1
  Err1/1 -> Mux/2
  Mux/1 -> human controller/1
  theta_ddot_des/1 -> Mux/3
  gravity accel/1 -> LEG gravity model/4(g)
  Tot mass/1 -> LEG gravity model/2(mLE)
  pos of CoM/1 -> LEG gravity model/3(LLE)
  Null TauH/1 -> Servo Control Enabler/1
  Null TauH1/1 -> Human Gravity Comp Enabler/1
  Human Gravity Comp Enabler/1 -> SumTauH/2
  SumTauH/1 -> Saturation/1
  human controller/1 -> Itot/1
  Servo Control Enabler/1 -> SumTauH/1
  Saturation/1 -> Tau_h/1
  Itot/1 -> Servo Control Enabler/2
  Null TauH2/1 -> Robot Torque Feedback/1
  TauR/1 -> Robot Torque Feedback/2
  Robot Torque Feedback/1 -> SumTauH/3
  theta/1 -> ROBOT gravity model/4(theta), LEG gravity model/1(theta), Err/2
  ROBOT gravity model/1(TauG_R) -> GravSum/2
  cost2/1 -> ROBOT gravity model/3(LR)
  cost/1 -> ROBOT gravity model/1(mR)
  cost1/1 -> ROBOT gravity model/2(g)
  LEG gravity model/1(TauG_h) -> GravSum/1
  GravSum/1 -> Human Gravity Comp Enabler/2

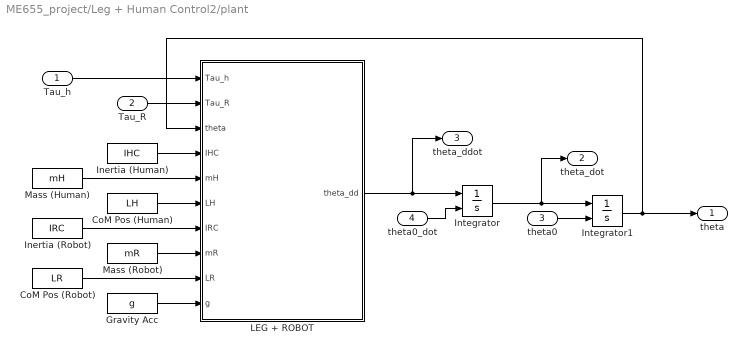
== system ME655_project/Leg + Human Control2/plant ==
  Tau_h : Inport
  Tau_R : Inport  Port=2
  theta0 : Inport  Port=3
  theta0_dot : Inport  Port=4
  CoM Pos (Human) : Constant  Value=LH
  CoM Pos (Robot) : Constant  Value=LR
  Gravity Acc : Constant  Value=g
  Inertia (Human) : Constant  Value=IHC
  Inertia (Robot) : Constant  Value=IRC
  Integrator : Integrator  InitialConditionSource=external  InitialCondition=theta_d0
  Integrator1 : Integrator  InitialConditionSource=external  InitialCondition=theta_0
  LEG + ROBOT : MATLAB Function  TreatAsAtomicUnit=on
  Mass (Human) : Constant  Value=mH
  Mass (Robot) : Constant  Value=mR
  theta : Outport  PortDimensions=[1,1]  VectorParamsAs1DForOutWhenUnconnected=off
  theta_dot : Outport  Port=2  PortDimensions=[1,1]  VectorParamsAs1DForOutWhenUnconnected=off
  theta_ddot : Outport  Port=3  PortDimensions=[1,1]  VectorParamsAs1DForOutWhenUnconnected=off
  wires:
  Tau_h/1 -> LEG + ROBOT/1(Tau_h)
  Tau_R/1 -> LEG + ROBOT/2(Tau_R)
  LEG + ROBOT/1(theta_dd) -> theta_ddot/1, Integrator/1
  Integrator/1 -> theta_dot/1, Integrator1/1
  theta0_dot/1 -> Integrator/2
  theta0/1 -> Integrator1/2
  Integrator1/1 -> LEG + ROBOT/3(theta), theta/1
  Inertia (Human)/1 -> LEG + ROBOT/4(IHC)
  Mass (Human)/1 -> LEG + ROBOT/5(mH)
  CoM Pos (Human)/1 -> LEG + ROBOT/6(LH)
  Gravity Acc/1 -> LEG + ROBOT/10(g)
  Mass (Robot)/1 -> LEG + ROBOT/8(mR)
  CoM Pos (Robot)/1 -> LEG + ROBOT/9(LR)
  Inertia (Robot)/1 -> LEG + ROBOT/7(IRC)

== matlab function ME655_project/Leg + Human Control2/human_motor_control/LEG gravity model ==
  data: theta input; mLE input; LLE input; TauG_h output; g input
function TauG_h   = HumanLegGravModel(theta,mLE,LLE,g)
% human gravity compensation term
TauG_h=mLE*g*LLE*sin(theta);

end

== matlab function ME655_project/Leg + Human Control/human_motor_control/LEG gravity model ==
  data: theta input; mLE input; LLE input; TauG_h output; g input
function TauG_h   = HumanLegGravModel(theta,mLE,LLE,g)
% human gravity compensation term
TauG_h=mLE*g*LLE*sin(theta);

end

== matlab function ME655_project/Leg + Human Control2/human_motor_control/ROBOT gravity model ==
  data: mR input; g input; LR input; theta input; TauG_R output
function TauG_R  = RobotGravModel(mR,g,LR,theta)

TauG_R=mR*g*LR*sin(theta);
% TauG_h=mLE*g*LLE*sin(theta);

end

== matlab function ME655_project/Tau_InverseDynamics2 ==
  data: theta_ddot input; Tau_tot output; theta input; IHC input; mH input; LH input; IRC input; mR input; LR input; g input
function Tau_tot = InverseDynamics(theta_ddot,theta,IHC,mH,LH,IRC,mR,LR,g)
Tau_tot = theta_ddot*((IRC + mR*LR^2)+(IHC + mH*LH^2)) + mH*g*LH*sin(theta) + mR*g*LR*sin(theta);

== matlab function ME655_project/Leg + Human Control/human_motor_control/ROBOT gravity model ==
  data: mR input; g input; LR input; theta input; TauG_R output
function TauG_R  = RobotGravModel(mR,g,LR,theta)

TauG_R=mR*g*LR*sin(theta);
% TauG_h=mLE*g*LLE*sin(theta);

end

== matlab function ME655_project/Leg + Human Control1/plant/LEG + ROBOT ==
  data: Tau_h input; Tau_R input; theta input; theta_dd output; IHC input; mH input; LH input; IRC input; mR input; LR input; g input
function theta_dd   = LegRobotModel(Tau_h,Tau_R,theta,IHC,mH,LH,IRC,mR,LR,g)

theta_dd = 1/((IRC + mR*LR^2)+(IHC + mH*LH^2)) * (Tau_h-mH*g*LH*sin(theta) + Tau_R-mR*g*LR*sin(theta));

end

== matlab function ME655_project/Leg + Human Control/plant/LEG + ROBOT ==
  data: Tau_h input; Tau_R input; theta input; theta_dd output; IHC input; mH input; LH input; IRC input; mR input; LR input; g input
function theta_dd   = LegRobotModel(Tau_h,Tau_R,theta,IHC,mH,LH,IRC,mR,LR,g)

theta_dd = 1/((IRC + mR*LR^2)+(IHC + mH*LH^2)) * (Tau_h-mH*g*LH*sin(theta) + Tau_R-mR*g*LR*sin(theta));

end

== matlab function ME655_project/Leg + Human Control2/plant/LEG + ROBOT ==
  data: Tau_h input; Tau_R input; theta input; theta_dd output; IHC input; mH input; LH input; IRC input; mR input; LR input; g input
function theta_dd   = LegRobotModel(Tau_h,Tau_R,theta,IHC,mH,LH,IRC,mR,LR,g)

theta_dd = 1/((IRC + mR*LR^2)+(IHC + mH*LH^2)) * (Tau_h-mH*g*LH*sin(theta) + Tau_R-mR*g*LR*sin(theta));

end

== matlab function ME655_project/CLME ==
  data: Rhip_pos_des input; Rhip_vel_des input; K input; k input; Lhip_pos_pred output; Lhip_vel_pred output
function [Lhip_pos_pred, Lhip_vel_pred] = generateLhipTrajectory(Rhip_pos_des, Rhip_vel_des, K, k)
    % Combine Rhip position and velocity into a matrix
    Rhip_des_data = [Rhip_pos_des, Rhip_vel_des];

    % Apply the CLME transformation using the trained parameters
    Lhip_pred = (K * Rhip_des_data' + k)';

    % Extract Lhip position and velocity from the result
    Lhip_pos_pred = Lhip_pred(:, 1);
    Lhip_vel_pred = Lhip_pred(:, 2);
end

== matlab function ME655_project/MATLAB Function ==
  data: theta input; theta_hat output; M input; eps input; nu input; dt input; AFO_ON input; state_in input; theta_dot_hat output; theta_ddot_hat output; Phi_1 output; state_out output
function [theta_hat, theta_dot_hat, theta_ddot_hat, Phi_1, state_out] = AFO(theta, M, eps, nu, dt, AFO_ON, state_in)
    Phi = state_in(1:6);
    a = state_in(7:12);
    w = state_in(13);
    theta0 = state_in(14);

    if AFO_ON == 0 
        state_out = state_in;
        theta_hat = 0;
        theta_dot_hat = 0;
        theta_ddot_hat = 0;
        Phi_1 = state_in(1);
    else
        % Update Oscillator State
        theta_next = theta - w * sum(a .* sin(Phi)) * dt - sum((1:M) .* w .* a .* cos(Phi)) * dt;

        % Update estimates of theta_dot and theta_ddot
        theta_dot_est = sum((1:M) .* w .* a .* cos(Phi));
        theta_ddot_est = -sum((1:M) .* w.^2 .* a .* sin(Phi));

        % Update Oscillator Parameters
        Phi = mod(Phi + dt * ((1:M) * w + eps * (theta - theta0 - sum(a .* sin(Phi))) * cos(Phi)), 2 * pi);
        a = a + dt * nu * (theta - theta0 - sum(a .* sin(Phi))) * sin(Phi);
        w = w + dt * eps * (theta - theta0 - sum(a .* sin(Phi))) * cos(Phi(1));
        theta0 = theta0 + dt * nu * (theta - theta0 - sum(a .* sin(Phi)));

        state_out = [Phi, a, w, theta0];

        % Output
        Phi_1 = Phi(1);
        theta_hat = theta_next;
        theta_dot_hat = theta_dot_est;
        theta_ddot_hat = theta_ddot_est;
    end
end

== matlab function ME655_project/Tau_InverseDynamics ==
  data: theta_ddot input; Tau_tot output; theta input; IHC input; mH input; LH input; IRC input; mR input; LR input; g input
function Tau_tot = InverseDynamics(theta_ddot,theta,IHC,mH,LH,IRC,mR,LR,g)
Tau_tot = theta_ddot*((IRC + mR*LR^2)+(IHC + mH*LH^2)) + mH*g*LH*sin(theta) + mR*g*LR*sin(theta);

== matlab function ME655_project/MATLAB Function1 ==
  data: Tau_tot input; Tau_R output; Ctrl_On input
function Tau_R = fcn(Tau_tot, Ctrl_On)
if Ctrl_On == 0
    Tau_R = 0;
else
    Tau_R = 0.5*Tau_tot;
end

== matlab function ME655_project/Kalman Filter ==
  data: A input; Lhip_pos_des output; Q input; R input; H input; Lhip_pos input; Lhip_vel input; xk_prev input; Pk_prev input; Lhip_vel_des output; xk_nxt output; Pk_nxt output
function [Lhip_pos_des, Lhip_vel_des, xk_nxt, Pk_nxt] = KF(A,Q,R,H,Lhip_pos,Lhip_vel,xk_prev,Pk_prev)
    
    zk = [Lhip_pos;Lhip_vel];
    %prediction stage
    xk_pred = A*xk_prev;
    Pk_pred = A*Pk_prev*A' + Q;
    
    %correction stage
    K = Pk_pred*H'*inv(H*Pk_pred*H' + R);
    xk_nxt = xk_pred + K*(zk - H*xk_prev);
    Pk_nxt = (eye(2) - K*H)*Pk_pred;

    Lhip_pos_des = xk_nxt(1);
    Lhip_vel_des = xk_nxt(2);
end

== matlab function ME655_project/Leg + Human Control1/human_motor_control/LEG gravity model ==
  data: theta input; mLE input; LLE input; TauG_h output; g input
function TauG_h   = HumanLegGravModel(theta,mLE,LLE,g)
% human gravity compensation term
TauG_h=mLE*g*LLE*sin(theta);

end

== matlab function ME655_project/Leg + Human Control1/human_motor_control/ROBOT gravity model ==
  data: mR input; g input; LR input; theta input; TauG_R output
function TauG_R  = RobotGravModel(mR,g,LR,theta)

TauG_R=mR*g*LR*sin(theta);
% TauG_h=mLE*g*LLE*sin(theta);

end

== matlab function ME655_project/NonLinearFilter ==
  data: AFO_ON input; est output; meas input; phi input; lambda input; N input; h input; P_in input; W_in input; P_out output; W_out output
function [est,P_out,W_out]= non_lin_filter(AFO_ON, meas, phi, lambda, N,h, P_in, W_in)

if AFO_ON == 0
    est = 0;
    P_out = P_in;
    W_out = W_in;
else
i=1;
est = 0;
est_num = 0;
est_den = 0;
P_out = P_in;
W_out = W_in;
while i <= N

    psi_i = exp(h*(cos(phi-((2*pi*i)/N))-1));


    %RLS
    e = meas-W_in;
    P_out = (1/lambda)*(P_in-((P_in^2)/((lambda/psi_i)+P_in)));
    W_out = W_in+psi_i*P_out*e;

    est_num = est_num + (psi_i*W_out);
    est_den = est_den + psi_i;
    est = est_num/est_den;
    i=i+1;

end
end
